simulink model "A421_FP_pt3_model"  (R2022b)
settings: Solver=VariableStepAuto  StartTime=0.0  StopTime=detumble.deltaT  RelTol=1e-3
undefined symbols (not defined in the file or in its folder): detumble
settings Model: Creator=willb  LastModifiedBy=willb

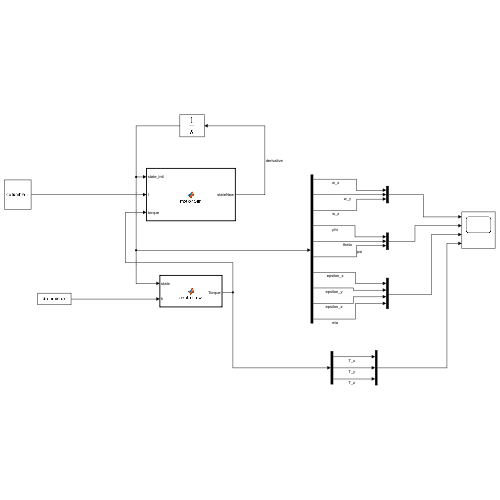
[thumbnail: Simulink's stored preview of the top-level diagram]
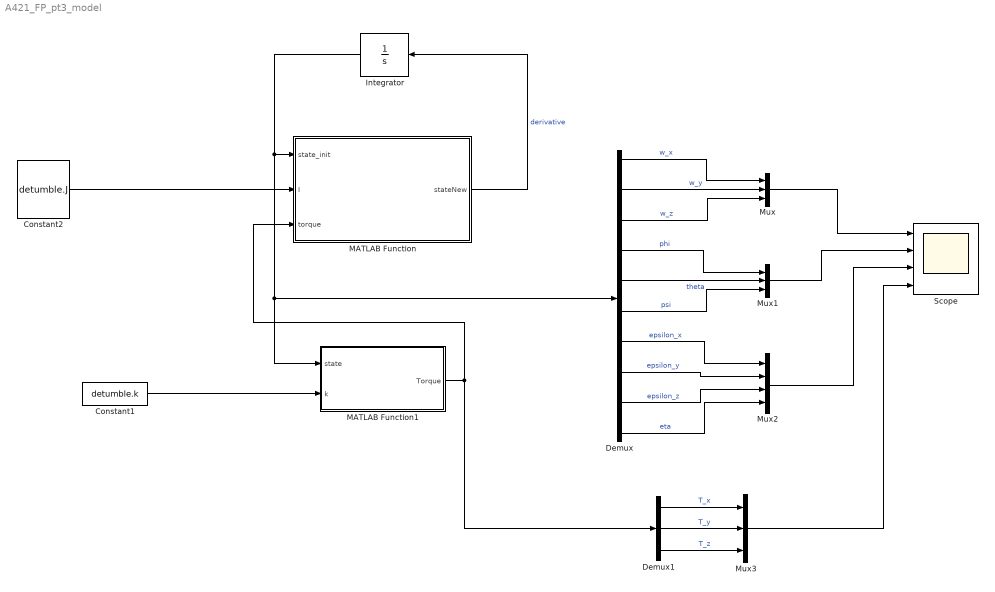
== system A421_FP_pt3_model ==
  Constant1 : Constant  Value=detumble.k
  Constant2 : Constant  Value=detumble.J
  Demux : Demux  Outputs=10
  Demux1 : Demux  Outputs=3
  Integrator : Integrator  InitialCondition=detumble.initialState
  MATLAB Function : MATLAB Function  TreatAsAtomicUnit=on
  MATLAB Function1 : MATLAB Function  TreatAsAtomicUnit=on
  Mux : Mux  Inputs=3
  Mux1 : Mux  Inputs=3
  Mux2 : Mux
  Mux3 : Mux  Inputs=3
  Scope : Scope  NumInputPorts=4
  wires:
  Integrator/1 -> MATLAB Function1/1(state), Demux/1, MATLAB Function/1(state_init)
  MATLAB Function/1(stateNew) -> Integrator/1  "derivative"
  Demux/2 -> Mux/2  "w_y"
  Mux1/1 -> Scope/2
  Mux/1 -> Scope/1
  Constant2/1 -> MATLAB Function/2(I)
  Demux/8 -> Mux2/2  "epsilon_y"
  Mux2/1 -> Scope/3
  Demux/3 -> Mux/3  "w_z"
  Demux/1 -> Mux/1  "w_x"
  Demux/5 -> Mux1/2  "theta"
  Demux/10 -> Mux2/4  "eta"
  Demux/9 -> Mux2/3  "epsilon_z"
  Demux/7 -> Mux2/1  "epsilon_x"
  Demux/6 -> Mux1/3  "psi"
  Demux/4 -> Mux1/1  "phi"
  MATLAB Function1/1(Torque) -> Demux1/1, MATLAB Function/3(torque)
  Constant1/1 -> MATLAB Function1/2(k)
  Demux1/2 -> Mux3/2  "T_y"
  Demux1/1 -> Mux3/1  "T_x"
  Demux1/3 -> Mux3/3  "T_z"
  Mux3/1 -> Scope/4

== matlab function A421_FP_pt3_model/MATLAB Function1 ==
  data: state input; Torque output; k input
function Torque  = controlLaw(state,k)

w = state(1:3);
Torque = -k*w;

== matlab function A421_FP_pt3_model/MATLAB Function ==
  data: stateNew output; state_init input; I input; torque input
function stateNew  = motionSim(state_init,I,torque)
% Inputs
    % time
    % state init = [wx,wy,wz,phi,theta,psi,epsilonx,epsilony,epsilonz,eta]
    % I = inertia matrix
    % torque
% Ouput
    % stateNew = derivative of stateInit
% *All angles in RADIANS*

% Angular Velocity
w_init = state_init(1:3);    
wx = w_init(1);
wy = w_init(2);
wz = w_init(3);
wcross = [0, -wz, wy; wz, 0, -wx; -wy, wx, 0];

% w_dot = (I^-1)*(-wcross*I*w_init+torque);
w_dot = (I^-1)*(torque-wcross*I*w_init);

% Euler Angles
initEuler = state_init(4:6);
phi = initEuler(1);
theta = initEuler(2);
psi = initEuler(3);

[Euler_dot] = (1/cos(theta))*...
    [cos(theta), sin(phi)*sin(theta), cos(phi)*sin(theta);...
     0,          cos(phi)*cos(theta), -sin(phi)*cos(theta);...
     0,          sin(phi), cos(phi)]*w_init;

% Quaternion
epsilon0 = state_init(7:9);
eta0 = state_init(10);
epsilCross = [          0, -epsilon0(3),  epsilon0(2); ...
              epsilon0(3),            0, -epsilon0(1); ...
             -epsilon0(2),  epsilon0(1),            0];

epsilonDot = 0.5*(eta0*eye(3) + epsilCross)*w_init;
etaDot = -0.5*epsilon0'*w_init;

stateNew = [w_dot;Euler_dot;epsilonDot;etaDot];
end
